simulink model "slotineParametrosIdentificados"  (R2014b)
settings: Solver=ode45  StartTime=0.0  StopTime=10.0  MaxStep=0.1  RelTol=1e-3
undefined symbols (not defined in the file): a, alpha, b, lambda
settings Model: Creator=roberto  LastModifiedBy=roberto

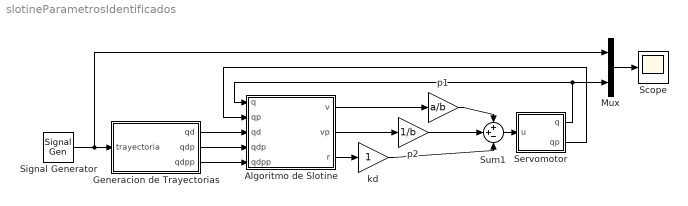
== system slotineParametrosIdentificados ==
  Algoritmo de Slotine : Subsystem
  Generacion de Trayectorias : Subsystem
  Mux : Mux  Inputs=2
  Scope : Scope
  Servomotor : Subsystem
  Signal Generator : SignalGenerator  Amplitude=0.5  Frequency=0.25
  Sum1 : Sum  Inputs=++-
  kd : Gain
  p1 : Gain  Gain=a/b
  p2 : Gain  Gain=1/b
  wires:
  Mux/1 -> Scope/1
  Signal Generator/1 -> Mux/1, Generacion de Trayectorias/1(trayectoria)
  Generacion de Trayectorias/1(qd) -> Algoritmo de Slotine/3(qd)
  Generacion de Trayectorias/2(qdp) -> Algoritmo de Slotine/4(qdp)
  Generacion de Trayectorias/3(qdpp) -> Algoritmo de Slotine/5(qdpp)
  Sum1/1 -> Servomotor/1(u)
  Servomotor/1(q) -> Mux/2, Algoritmo de Slotine/1(q)
  Servomotor/2(qp) -> Algoritmo de Slotine/2(qp)
  Algoritmo de Slotine/2(vp) -> p2/1
  p2/1 -> Sum1/2
  Algoritmo de Slotine/1(v) -> p1/1
  p1/1 -> Sum1/1
  kd/1 -> Sum1/3
  Algoritmo de Slotine/3(r) -> kd/1

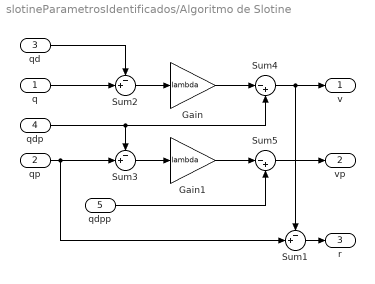
== system slotineParametrosIdentificados/Algoritmo de Slotine ==
  q : Inport
  qp : Inport  Port=2
  qd : Inport  Port=3
  qdp : Inport  Port=4
  qdpp : Inport  Port=5
  Gain : Gain  Gain=lambda
  Gain1 : Gain  Gain=lambda
  Sum1 : Sum  Inputs=-+|
  Sum2 : Sum  Inputs=-+|
  Sum3 : Sum  Inputs=-+|
  Sum4 : Sum  Inputs=|-+
  Sum5 : Sum  Inputs=|-+
  v : Outport
  vp : Outport  Port=2
  r : Outport  Port=3
  wires:
  Gain/1 -> Sum4/1
  qp/1 -> Sum1/2, Sum3/2
  Sum4/1 -> Sum1/1, v/1
  q/1 -> Sum2/2
  Sum5/1 -> vp/1
  Sum3/1 -> Gain1/1
  Gain1/1 -> Sum5/1
  Sum2/1 -> Gain/1
  qdpp/1 -> Sum5/2
  qdp/1 -> Sum3/1, Sum4/2
  qd/1 -> Sum2/1
  Sum1/1 -> r/1

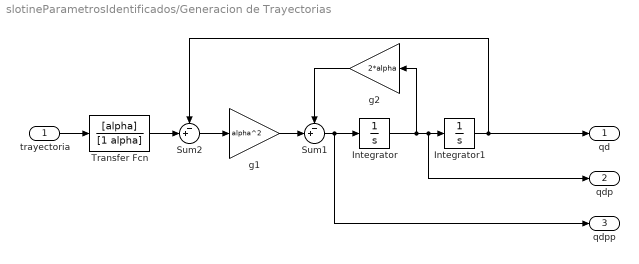
== system slotineParametrosIdentificados/Generacion de Trayectorias ==
  trayectoria : Inport
  Integrator : Integrator
  Integrator1 : Integrator
  Sum1 : Sum  Inputs=-+|
  Sum2 : Sum  Inputs=-+|
  Transfer Fcn : TransferFcn  Numerator=[alpha]  Denominator=[1 alpha]
  g1 : Gain  Gain=alpha^2
  g2 : Gain  Gain=2*alpha
  qd : Outport
  qdp : Outport  Port=2
  qdpp : Outport  Port=3
  wires:
  Sum2/1 -> g1/1
  trayectoria/1 -> Transfer Fcn/1
  Integrator1/1 -> qd/1, Sum2/1
  Integrator/1 -> g2/1, qdp/1, Integrator1/1
  g1/1 -> Sum1/2
  Sum1/1 -> qdpp/1, Integrator/1
  g2/1 -> Sum1/1
  Transfer Fcn/1 -> Sum2/2

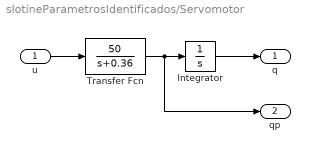
== system slotineParametrosIdentificados/Servomotor ==
  u : Inport
  Integrator : Integrator
  Transfer Fcn : TransferFcn  Numerator=[50]  Denominator=[1 0.36]
  q : Outport
  qp : Outport  Port=2
  wires:
  Transfer Fcn/1 -> Integrator/1, qp/1
  u/1 -> Transfer Fcn/1
  Integrator/1 -> q/1
